simulink model "noises"  (Simulink 7.1)
settings: Solver=ode45  StartTime=0.0  StopTime=noisessimtime  MaxStep=tr_noises  RelTol=1e-3
values from neighbouring files (symbols this model uses):
  dens = [M B k]    [mechanical_example.m]
  nums = [B k]    [mechanical_example.m]
settings Model: Creator=christopher.rappa  LastModifiedBy=christopher.rappa
settings OptimizationCC: InlineInvariantSignals=on
settings DebuggingCC: SaveWithParameterizedLinksMsg=none  SignalResolutionControl=TryResolveAllWithWarning  MultiTaskDSMMsg=warning  MultiTaskCondExecSysMsg=none  StrictBusMsg=None
settings RTWCC: IncludeERTFirstTime=on
settings GRTTargetCC: TargetFcnLib=ansi_tfl_tmw.mat

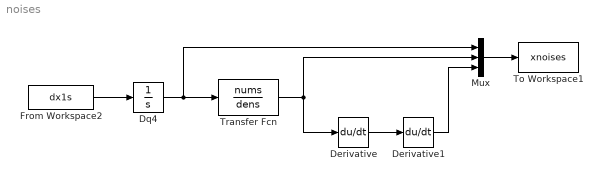
== system noises ==
  Derivative : Derivative
  Derivative1 : Derivative
  Dq4 : Integrator
  From Workspace2 : FromWorkspace  VariableName=dx1s  SampleTime=0
  Mux : Mux  Inputs=3
  To Workspace1 : ToWorkspace  VariableName=xnoises  SampleTime=-1  SaveFormat=Structure With Time
  Transfer Fcn : TransferFcn  Numerator=nums  Denominator=dens
  wires:
  Dq4/1 -> Mux/1, Transfer Fcn/1
  From Workspace2/1 -> Dq4/1
  Mux/1 -> To Workspace1/1
  Transfer Fcn/1 -> Mux/2, Derivative/1
  Derivative/1 -> Derivative1/1
  Derivative1/1 -> Mux/3
